simulink model "C172S_LateralDirectionalPlant_V01"  (R2026a)
settings: Solver=ode4  StartTime=0  StopTime=20  FixedStep=0.01
InitFcn:
  | ldpData = c172sLateralDirectionalData();
  | [~,ldpPlant] = c172sLateralDirectionalPlant(ldpData);
  | A_ldp = ldpPlant.A; B_ldp = ldpPlant.B;
  | C_ldp = ldpPlant.C; D_ldp = ldpPlant.D;
  | if ~exist('deltaACommand_ldp_rad','var'), deltaACommand_ldp_rad = deg2rad(1.0); end
  | if ~exist('deltaRCommand_ldp_rad','var'), deltaRCommand_ldp_rad = deg2rad(1.0); end
  | if ~exist('x0_ldp','var'), x0_ldp = zeros(5,1); end
undefined symbols (not defined in the file or in its folder): deltaACommand_ldp_rad, deltaRCommand_ldp_rad, x0_ldp
settings Model: Creator=Shahi  LastModifiedBy=Shahi

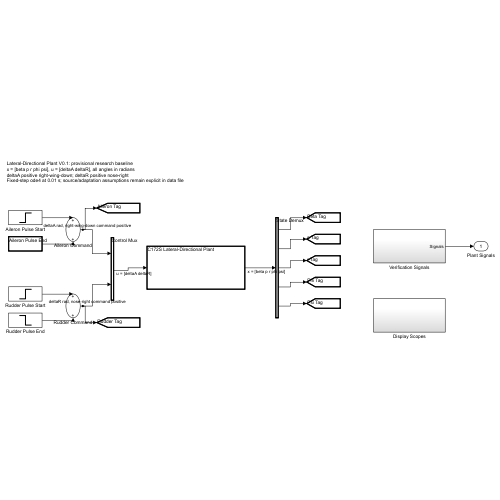
[thumbnail: Simulink's stored preview of the top-level diagram]
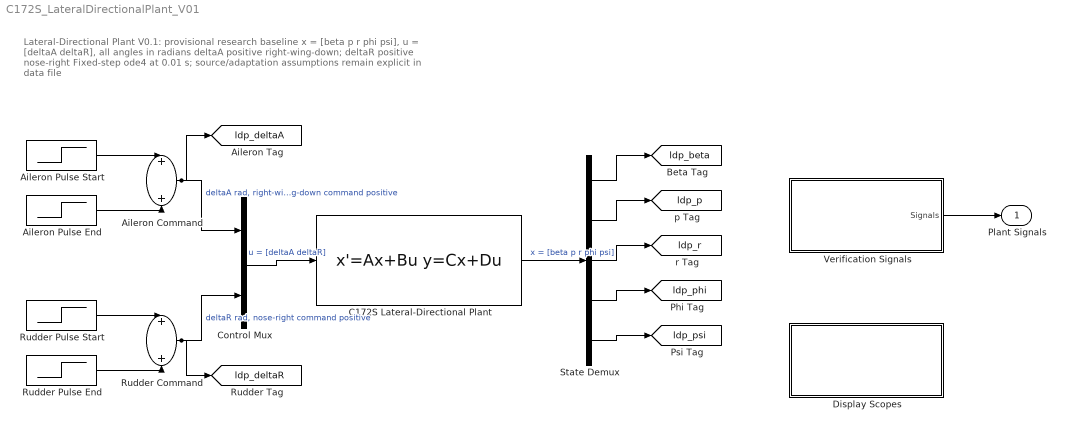
== system C172S_LateralDirectionalPlant_V01 ==
  note: Lateral-Directional Plant V0.1: provisional research baseline
      | x = [beta p r phi psi], u = [deltaA deltaR], all angles in radians
      | deltaA positive right-wing-down; deltaR positive nose-right
      | Fixed-step ode4 at 0.01 s; source/adaptation assumptions remain explicit in data file
  Aileron Command : Sum
  Aileron Pulse End : Step  FinalValue=-deltaACommand_ldp_rad  SampleTime=0
  Aileron Pulse Start : Step  Time=0  FinalValue=deltaACommand_ldp_rad  SampleTime=0
  C172S Lateral-Directional Plant : StateSpace  A=A_ldp  B=B_ldp  C=C_ldp  D=D_ldp  InitialCondition=x0_ldp
  Control Mux : Mux  Inputs=2
  Display Scopes : Subsystem
  Rudder Command : Sum
  Rudder Pulse End : Step  Time=6  FinalValue=-deltaRCommand_ldp_rad  SampleTime=0
  Rudder Pulse Start : Step  Time=5  FinalValue=deltaRCommand_ldp_rad  SampleTime=0
  State Demux : Demux  Outputs=5
  Verification Signals : Subsystem
  Plant Signals : Outport
  tag scope: ldp_beta=global, ldp_deltaA=global, ldp_deltaR=global, ldp_p=global, ldp_phi=global, ldp_psi=global, ldp_r=global
  wires:
  Verification Signals/1(Signals) -> Plant Signals/1
  Aileron Pulse Start/1 -> Aileron Command/1
  Aileron Pulse End/1 -> Aileron Command/2
  Rudder Pulse Start/1 -> Rudder Command/1
  Rudder Pulse End/1 -> Rudder Command/2
  Aileron Command/1 -> Control Mux/1, [ldp_deltaA]  "deltaA rad, right-wing-down command positive"
  Rudder Command/1 -> Control Mux/2, [ldp_deltaR]  "deltaR rad, nose-right command positive"
  Control Mux/1 -> C172S Lateral-Directional Plant/1  "u = [deltaA deltaR]"
  C172S Lateral-Directional Plant/1 -> State Demux/1  "x = [beta p r phi psi]"
  State Demux/1 -> [ldp_beta]
  State Demux/2 -> [ldp_p]
  State Demux/3 -> [ldp_r]
  State Demux/4 -> [ldp_phi]
  State Demux/5 -> [ldp_psi]

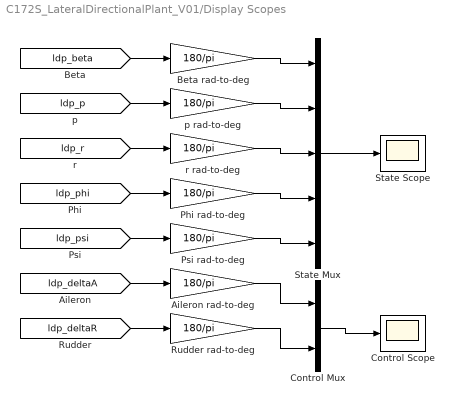
== system C172S_LateralDirectionalPlant_V01/Display Scopes ==
  Aileron rad-to-deg : Gain  Gain=180/pi
  Beta rad-to-deg : Gain  Gain=180/pi
  Control Mux : Mux  Inputs=2
  Control Scope : Scope
  Phi rad-to-deg : Gain  Gain=180/pi
  Psi rad-to-deg : Gain  Gain=180/pi
  Rudder rad-to-deg : Gain  Gain=180/pi
  State Mux : Mux  Inputs=5
  State Scope : Scope
  p rad-to-deg : Gain  Gain=180/pi
  r rad-to-deg : Gain  Gain=180/pi
  wires:
  [ldp_beta] -> Beta rad-to-deg/1
  [ldp_p] -> p rad-to-deg/1
  [ldp_r] -> r rad-to-deg/1
  [ldp_phi] -> Phi rad-to-deg/1
  [ldp_psi] -> Psi rad-to-deg/1
  [ldp_deltaA] -> Aileron rad-to-deg/1
  [ldp_deltaR] -> Rudder rad-to-deg/1
  Beta rad-to-deg/1 -> State Mux/1
  p rad-to-deg/1 -> State Mux/2
  r rad-to-deg/1 -> State Mux/3
  Phi rad-to-deg/1 -> State Mux/4
  Psi rad-to-deg/1 -> State Mux/5
  State Mux/1 -> State Scope/1
  Aileron rad-to-deg/1 -> Control Mux/1
  Rudder rad-to-deg/1 -> Control Mux/2
  Control Mux/1 -> Control Scope/1

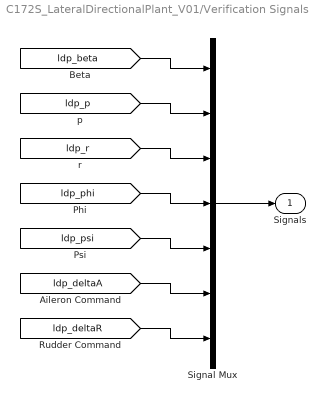
== system C172S_LateralDirectionalPlant_V01/Verification Signals ==
  Signal Mux : Mux  Inputs=7
  Signals : Outport
  wires:
  [ldp_beta] -> Signal Mux/1
  [ldp_p] -> Signal Mux/2
  [ldp_r] -> Signal Mux/3
  [ldp_phi] -> Signal Mux/4
  [ldp_psi] -> Signal Mux/5
  [ldp_deltaA] -> Signal Mux/6
  [ldp_deltaR] -> Signal Mux/7
  Signal Mux/1 -> Signals/1
